simulink model "pll_6"  (Simulink 2.20)
settings: Solver=ode45  StartTime=0.0  StopTime=10.0  RelTol=1e-3  AbsTol=1e-6
settings Model: ConsistencyChecking=off  RTWPlaceOutputsASAP=off

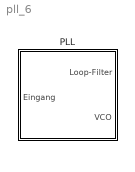
== system pll_6 ==
  PLL : Subsystem  mask(PLL-Schleife){f0=, ph_fehler=, kvco=, tau=}
      mask prompts: f0 "Ruhefrequenz"; ph_fehler "Phasenfehler-VCO"; kvco "Übertragungsfaktor-VCO"; tau "Zeitkonstante-Filter"
      mask help: Es wird eine analoge PLL-Schleife simuliert. Der Phasen-Detektor besteht aus einem Multiplizierer.
      mask init:
      | t = [0:0.1:2*pi,0];
      | x = cos(t);    y = sin(t);
      mask Help:
      | Pll-Schleife bestehend aus einem Multiplizierer als Phasen-Detektor, Tiefpaßfilter erster Ordnung und VCO. Die Parameter sind:
      | tau = Zeitkonstante des Filters
      | kvco = Übertragungsfaktor des VCOs
      | ph_fehler = Anfangsphasenfehler des VCO
      | f0 = Ruhefrequenz

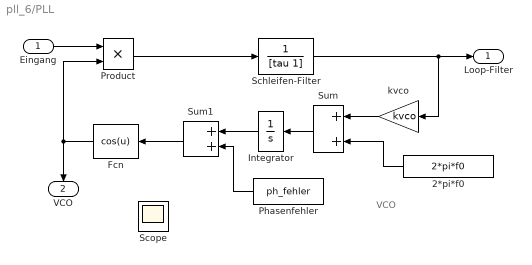
== system pll_6/PLL ==
  note: VCO
  Eingang : Inport  Port=1  PortWidth=-1  SampleTime=-1
  2*pi*f0 : Constant  Orientation=left  Value=2*pi*f0
  Fcn : Fcn  Orientation=left  Expr=cos(u)
  Integrator : Integrator  Orientation=left  ExternalReset=none  InitialConditionSource=internal  InitialCondition=0  LimitOutput=off  UpperSaturationLimit=inf  LowerSaturationLimit=-inf  ShowSaturationPort=off  ShowStatePort=off  AbsoluteTolerance=auto
  Phasenfehler : Constant  Orientation=left  Value=ph_fehler
  Product : Product  Inputs=2
  Schleifen-Filter : TransferFcn  Numerator=[1]  Denominator=[tau 1]
  Scope : Scope
      settings: Floating=on  TickLabels=on  TimeRange=0.1  YMin=-5  YMax=5  SaveToWorkspace=off  SaveName=ScopeData
  Sum : Sum  Orientation=left  Inputs=++
  Sum1 : Sum  Orientation=left  Inputs=++
  kvco : Gain  Orientation=left  Gain=kvco
  Loop-Filter : Outport  Port=1  InitialOutput=0
  " VCO" : Outport  Orientation=down  Port=2  InitialOutput=0
  wires:
  Integrator/1 -> Sum1/1
  Phasenfehler/1 -> Sum1/2
  Schleifen-Filter/1 -> Loop-Filter/1, kvco/1
  kvco/1 -> Sum/1
  2*pi*f0/1 -> Sum/2
  Sum/1 -> Integrator/1
  Product/1 -> Schleifen-Filter/1
  Sum1/1 -> Fcn/1
  Eingang/1 -> Product/1
  Fcn/1 -> " VCO"/1, Product/2
